simulink model "es2_2_diagonals"  (R2024b)
settings: Solver=VariableStepAuto  StartTime=0.0  StopTime=30  RelTol=1e-3
libraries: sharedutil x1, vrlib x1
settings Model: Creator=danie  LastModifiedBy=danie

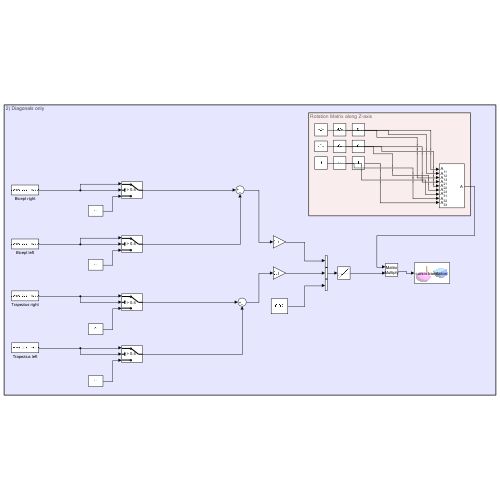
[thumbnail: Simulink's stored preview of the top-level diagram]
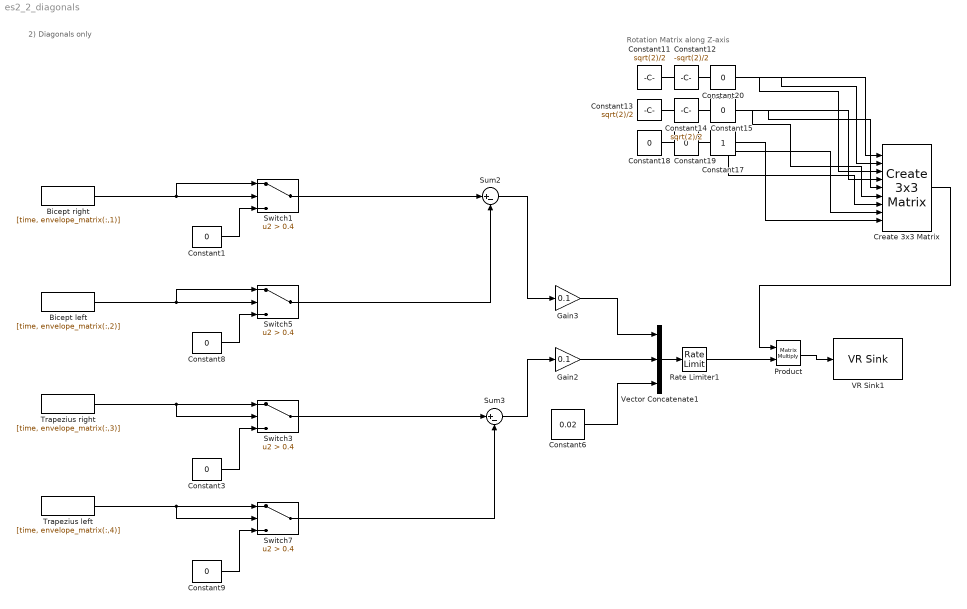
== system es2_2_diagonals ==
  note: 2) Diagonals only
  note: Rotation Matrix along Z-axis
  Bicept left : FromWorkspace  VariableName=[time, envelope_matrix(:,2)]
  Bicept right : FromWorkspace  VariableName=[time, envelope_matrix(:,1)]
  Constant{1,3,8..9,15,18..20} (8 alike) : Constant  Value=0
  Constant11 : Constant  Value=sqrt(2)/2
  Constant12 : Constant  Value=-sqrt(2)/2
  Constant13 : Constant  Value=sqrt(2)/2
  Constant14 : Constant  Value=sqrt(2)/2
  Constant17 : Constant
  Constant6 : Constant  Value=0.02
  Create 3x3 Matrix : sharedutil/Create 3x3 Matrix  aMode=aMode
      settings: LibrarySourceBlock=aerolibutil/Create 3x3 Matrix
  Gain2 : Gain  Gain=0.1
  Gain3 : Gain  Gain=0.1
  Product : Product  Multiplication=Matrix(*)
  Rate Limiter1 : RateLimiter  RisingSlewLimit=0.4  FallingSlewLimit=-0.4  SampleTimeMode=inherited
  Sum2 : Sum  Inputs=|+-
  Sum3 : Sum  Inputs=|+-
  Switch{1,3,5,7} (4 alike) : Switch  Criteria=u2 > Threshold  Threshold=0.4  SaturateOnIntegerOverflow=off  InputSameDT=off
  Trapezius left : FromWorkspace  VariableName=[time, envelope_matrix(:,4)]
  Trapezius right : FromWorkspace  VariableName=[time, envelope_matrix(:,3)]
  VR Sink1 : vrlib/VR Sink  InstantiateOnLoad=on  SampleTime=0.1  ViewEnable=on  RemoteChange=off  RemoteView=off  FieldsWritten=cursor.translation.3.1.1.double  WorldFileName=8_palline_color.wrl  AutoView=off  VideoDimensions=[]  AllowVariableSize=off
  Vector Concatenate1 : Concatenate  NumInputs=3
  wires:
  Bicept right/1 -> Switch1/2, Switch1/1
  Switch1/1 -> Sum2/1
  Constant15/1 -> Create 3x3 Matrix/6
  Constant1/1 -> Switch1/3
  Switch7/1 -> Sum3/2
  Create 3x3 Matrix/1 -> Product/1
  Switch3/1 -> Sum3/1
  Product/1 -> VR Sink1/1
  Constant3/1 -> Switch3/3
  Constant14/1 -> Create 3x3 Matrix/5
  Constant17/1 -> Create 3x3 Matrix/9
  Bicept left/1 -> Switch5/1, Switch5/2
  Gain2/1 -> Vector Concatenate1/2
  Constant12/1 -> Create 3x3 Matrix/2
  Constant13/1 -> Create 3x3 Matrix/4
  Rate Limiter1/1 -> Product/2
  Constant20/1 -> Create 3x3 Matrix/3
  Sum3/1 -> Gain2/1
  Trapezius right/1 -> Switch3/1, Switch3/2
  Constant11/1 -> Create 3x3 Matrix/1
  Constant18/1 -> Create 3x3 Matrix/7
  Constant8/1 -> Switch5/3
  Vector Concatenate1/1 -> Rate Limiter1/1
  Gain3/1 -> Vector Concatenate1/1
  Sum2/1 -> Gain3/1
  Constant6/1 -> Vector Concatenate1/3
  Switch5/1 -> Sum2/2
  Trapezius left/1 -> Switch7/1, Switch7/2
  Constant9/1 -> Switch7/3
  Constant19/1 -> Create 3x3 Matrix/8
